simulink model "exampleStorageTnodes"  (R2016b)
settings: Solver=ode45  StartTime=0.0  StopTime=3*3600  MaxStep=300  RelTol=1e-3  EnableMultiTasking=on
libraries: carnot x18
settings Model: Creator=drhf  LastModifiedBy=drhf
settings DataIOCC: LimitDataPoints=on  SaveFormat=Array  SignalLoggingSaveFormat=ModelDataLogs
settings OptimizationCC: ExpressionDepthLimit=2147483647  LifeSpan=inf
settings DebuggingCC: UnderspecifiedInitializationDetection=Classic  MergeDetectMultiDrivingBlocksExec=none  SolverPrmCheckMsg=warning  FcnCallInpInsideContextMsg=warning  StateNameClashWarn=warning  SFUnexpectedBacktrackingDiag=warning  SFNoUnconditionalDefaultTransitionDiag=warning  SFExecutionAtInitializationDiag=none
settings HardwareCC: ProdBitPerPointer=32  ProdBitPerSizeT=32  ProdBitPerPtrDiffT=32  ProdLargestAtomicFloat=None  ProdIntDivRoundTo=Undefined  ProdEndianess=Unspecified  ProdWordSize=32  ProdHWDeviceType=32-bit Generic
settings ModelReferenceCC: PropagateSignalLabelsOutOfModel=off
settings GRTTargetCC: TargetLangStandard=C89/C90 (ANSI)  GeneratePreprocessorConditionals=Disable all  CombineOutputUpdateFcns=off  GRTInterface=on
settings ConfigComp: CovMetricSettings=dw  CovHtmlReporting=on  CovSaveCumulativeToWorkspaceVar=on  CovSaveSingleToWorkspaceVar=on  CovExternalEMLEnable=off

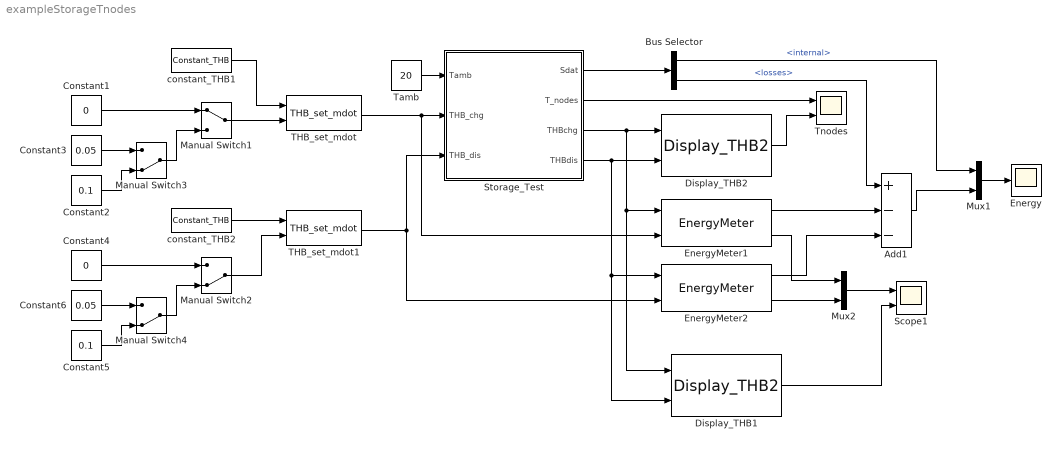
== system exampleStorageTnodes ==
  Add1 : Sum  Inputs=+--
  Bus Selector : BusSelector  OutputSignals=energy.internal,energy.losses
  Constant1 : Constant  Value=0
  Constant2 : Constant  Value=0.1
  Constant3 : Constant  Value=0.05
  Constant4 : Constant  Value=0
  Constant5 : Constant  Value=0.1
  Constant6 : Constant  Value=0.05
  Display_THB1 : carnot/Outputs/Display_THB2  t=on  m=off  p=off  id=off  mix=off  d=off
  Display_THB2 : carnot/Outputs/Display_THB2  t=off  m=on  p=off  id=off  mix=off  d=off
  Energy : Scope
  EnergyMeter1 : carnot/Control/EnergyMeter
  EnergyMeter2 : carnot/Control/EnergyMeter
  Manual Switch1 : ManualSwitch
  Manual Switch2 : ManualSwitch  CurrentSetting=0
  Manual Switch3 : ManualSwitch  CurrentSetting=0
  Manual Switch4 : ManualSwitch  CurrentSetting=0
  Mux1 : Mux  Inputs=2
  Mux2 : Mux  Inputs=2
  Scope1 : Scope  NumInputPorts=2
  Storage_Test : Subsystem  mask(Multiport Storage){uloss=0, ubot=0, utop=0, cond=0, t0=[10 10 55 55], volume=0.3, dia=0.5, nconnect=2, standing=standing cylinder, hgt=1.5279, nodes=10, mpoints=10}
      mask prompts: uloss "Heat loss coefficient cylinder wall in W/(m²K)"; ubot "Heat loss coefficient bottom in W/(m²K)"; utop "Heat loss coefficient top cover in W/(m²K)"; cond "Effective vertical conductivity in W/(m*K)"; t0 "Initial temperature (vector or scalar) in °C"; volume "Volume in m³"; dia "Diameter in m"; nconnect "Number of connections"; standing "Position"; hgt "Height of storage"; nodes "Number of nodes"; mpoints "Number of measurement points"
      mask help:
      | The volmue of the cylindrical storage is divided in a number "nodes" of horizontal slices (1xN-node model). For each node the energy balance equation is solved.
      | Look under mask to set the ports types and properties.
      mask init:
      | [~, dh, height, mpts, tini] ...
      |     = CarnotCallbacks_StorageTypeN(3-standing, volume, dia, nodes, mpoints, t0);
      | set_param(gcb,'hgt',num2str(height));
      | uloss
      | ubot
      | utop
      | cond
      | t0
      | volume
      | dia
      | height
      | hgt
      | nconnect
      | standing
      | nodes
      | mpoints
      mask Help: web(fullfile(path_carnot('help'),'storage_multiport.html'),'-helpbrowser')
      mask TypeOptions standing: sfun_storageTnodes/standing
      mask Display: plot(10,10,90,100,[40,40,45,55,60,60,55,45,40],[84,36,30,30,36,84,90,90,84],[40,35],[77,77],[64,60],[77,77],[40,35],[42,42],[64,60],[42,42])
  THB_set_mdot : carnot/Source/Simple/THB_set_mdot
  THB_set_mdot1 : carnot/Source/Simple/THB_set_mdot
  Tamb : Constant  Value=20
  Tnodes : Scope  NumInputPorts=2
  constant_THB1 : carnot/Source/Simple/Constant_THB  t=55  mdot=0*100/3600  p=1e5  mID=Full Pressure Drop with Static Height  fluid=Water  mix=0  mix2=0  mix3=0  dia=0.02  hgt=0
  constant_THB2 : carnot/Source/Simple/Constant_THB  t=10  mdot=100/3600  p=1e5  mID=Full Pressure Drop with Static Height  fluid=Water  mix=0  mix2=0  mix3=0  dia=0.02  hgt=0
  wires:
  Bus Selector/1 -> Mux1/1  "<internal>"
  Tamb/1 -> Storage_Test/1(Tamb)
  THB_set_mdot/1 -> EnergyMeter1/2, Storage_Test/2(THB_chg)
  THB_set_mdot1/1 -> Storage_Test/3(THB_dis), EnergyMeter2/2
  Storage_Test/1(Sdat) -> Bus Selector/1
  Storage_Test/2(T_nodes) -> Tnodes/1
  Storage_Test/3(THBchg) -> Display_THB2/1, EnergyMeter1/1, Display_THB1/1
  Storage_Test/4(THBdis) -> Display_THB2/2, EnergyMeter2/1, Display_THB1/2
  Display_THB2/1 -> Tnodes/2
  Mux1/1 -> Energy/1
  EnergyMeter2/2 -> Mux2/2
  constant_THB1/1 -> THB_set_mdot/1
  constant_THB2/1 -> THB_set_mdot1/1
  Manual Switch1/1 -> THB_set_mdot/2
  Manual Switch2/1 -> THB_set_mdot1/2
  Constant1/1 -> Manual Switch1/1
  EnergyMeter1/2 -> Mux2/1
  Add1/1 -> Mux1/2
  EnergyMeter2/1 -> Add1/3
  EnergyMeter1/1 -> Add1/2
  Bus Selector/2 -> Add1/1  "<losses>"
  Constant3/1 -> Manual Switch3/1
  Manual Switch3/1 -> Manual Switch1/2
  Constant2/1 -> Manual Switch3/2
  Constant4/1 -> Manual Switch2/1
  Constant6/1 -> Manual Switch4/1
  Manual Switch4/1 -> Manual Switch2/2
  Constant5/1 -> Manual Switch4/2
  Mux2/1 -> Scope1/1
  Display_THB1/1 -> Scope1/2

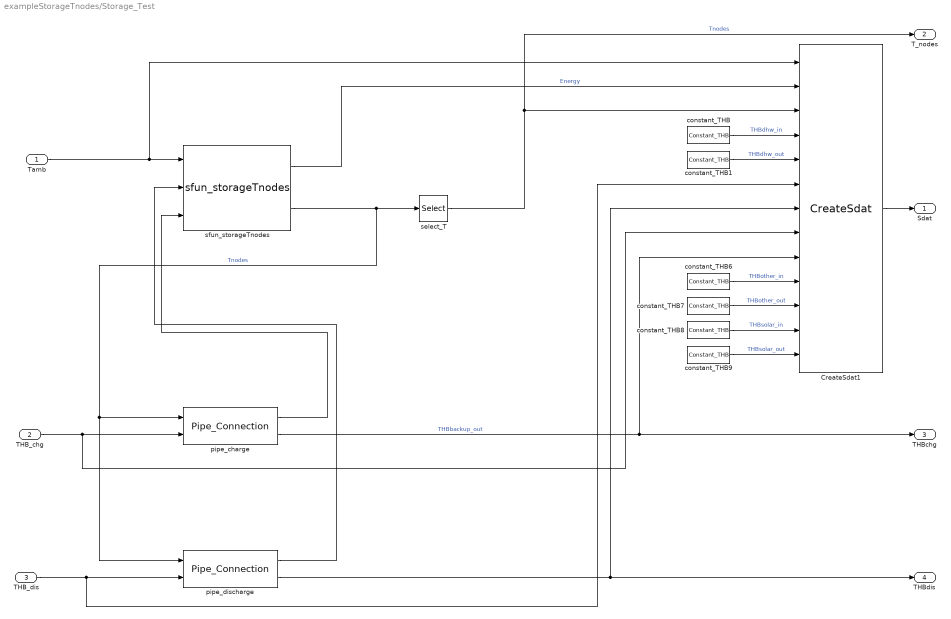
== system exampleStorageTnodes/Storage_Test ==
  Tamb : Inport
  THB_chg : Inport  Port=2
  THB_dis : Inport  Port=3
  CreateSdat1 : carnot/Basic/Thermal_Models/CreateSdat  volume=0.1
  constant_THB{,1,6..9} (6 alike) : carnot/Source/Simple/Constant_THB  t=20  mdot=0  p=1e5  mID=No Pressure Drop  fluid=Water  mix=0  mix2=0  mix3=0  dia=0.02  hgt=0
  pipe_charge : carnot/Storage/Thermal/Storage_Ports/Pipe_Connection  h_in=0.8  h_out=0.2  hgt=height  dia=dia  height=-0.91673  nodes=nodes
  pipe_discharge : carnot/Storage/Thermal/Storage_Ports/Pipe_Connection  h_in=0.2  h_out=0.8  hgt=height  dia=dia  height=0.91673  nodes=nodes
  select_T : Selector  InputPortWidth=nodes  IndexOptions=Index vector (dialog)  Indices=mpts  OutputSizes=1
  sfun_storageTnodes : carnot/Basic/Thermal_Models/sfun_storageTnodes  uloss=uloss  ubot=utop  utop=ubot  cond=cond  volume=volume  dia=dia  standing=standing cylinder  tini=tini  nodes=nodes  nconnect=nconnect  elimthermocline=1  condinvtc=1e5
  Sdat : Outport
  T_nodes : Outport  Port=2
  THBchg : Outport  Port=3
  THBdis : Outport  Port=4
  wires:
  pipe_charge/1 -> sfun_storageTnodes/3
  pipe_charge/2 -> CreateSdat1/9, THBchg/1  "THBbackup_out"
  THB_chg/1 -> CreateSdat1/8, pipe_charge/2
  sfun_storageTnodes/2 -> pipe_discharge/1, pipe_charge/1, select_T/1  "Tnodes"
  sfun_storageTnodes/1 -> CreateSdat1/2  "Energy"
  select_T/1 -> T_nodes/1, CreateSdat1/3  "Tnodes"
  pipe_discharge/1 -> sfun_storageTnodes/2
  pipe_discharge/2 -> CreateSdat1/7, THBdis/1
  THB_dis/1 -> CreateSdat1/6, pipe_discharge/2
  Tamb/1 -> CreateSdat1/1, sfun_storageTnodes/1
  constant_THB/1 -> CreateSdat1/4  "THBdhw_in"
  constant_THB1/1 -> CreateSdat1/5  "THBdhw_out"
  constant_THB6/1 -> CreateSdat1/10  "THBother_in"
  constant_THB7/1 -> CreateSdat1/11  "THBother_out"
  constant_THB8/1 -> CreateSdat1/12  "THBsolar_in"
  constant_THB9/1 -> CreateSdat1/13  "THBsolar_out"
  CreateSdat1/1 -> Sdat/1
